simulink model "LQRAirrefuelingYingHu_full2Model"  (R2013a)
settings: Solver=ode45  StartTime=0.0  StopTime=100  RelTol=1e-3
values from neighbouring files (symbols this model uses):
  A_full = [A_full(1:7,1:7),zeros(7,1),A_full(1:7,8:11) ... (first row only)    [LQR_Calc2_F16YingHu_lonAndLa.m]
  B_full = [zeros(1,4);B(1:6,1:4);zeros(1,4);B(7:10,1:4)]    [LQR_Calc2_F16YingHu_lonAndLa.m]
  C_xd_h_yd = [C_xd_h,zeros(2,5) ... (first row only)    [LQR_Calc2_F16YingHu_lonAndLa.m]
  Ki = [Ki_lon,zeros(2,1) ... (first row only)    [LQR_Calc2_F16YingHu_lonAndLa.m]
  Kp = [Kp_lon,zeros(2,5) ... (first row only)    [LQR_Calc2_F16YingHu_lonAndLa.m]
undefined symbols (not defined in the file or in its folder): W_full
libraries: simulink x3
settings Model: Creator=Dai  LastModifiedBy=Dai

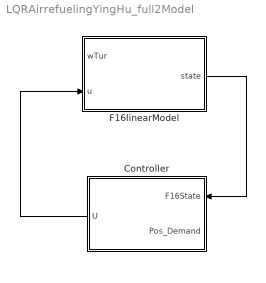
== system LQRAirrefuelingYingHu_full2Model ==
  Controller : Subsystem
  F16linearModel : Subsystem
  wires:
  F16linearModel/1(state) -> Controller/1(F16State)
  Controller/1(U) -> F16linearModel/2(u)

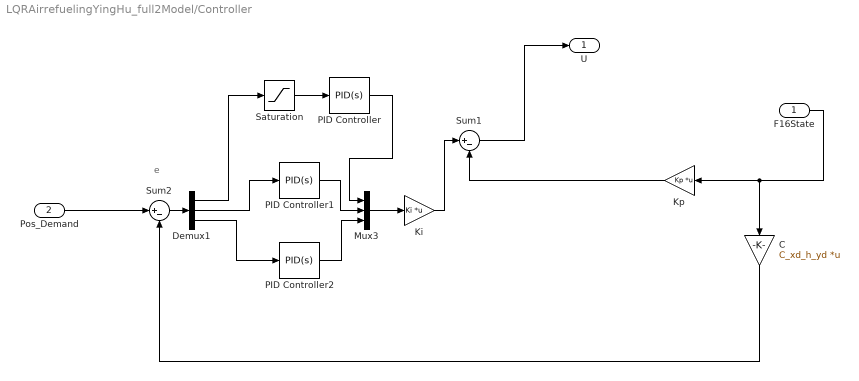
== system LQRAirrefuelingYingHu_full2Model/Controller ==
  note: e
  F16State : Inport
  Pos_Demand : Inport  Port=2
  C : Gain  Gain=C_xd_h_yd  Multiplication=Matrix(K*u) (u vector)
  Demux1 : Demux  Outputs=3
  Ki : Gain  Gain=Ki  Multiplication=Matrix(K*u) (u vector)
  Kp : Gain  Gain=Kp  Multiplication=Matrix(K*u) (u vector)
  Mux3 : Mux  Inputs=3
  PID Controller : simulink/Continuous/PID Controller  Controller=PID  TimeDomain=Continuous-time  SampleTime=1  IntegratorMethod=Forward Euler  FilterMethod=Forward Euler  Form=Parallel  P=0  I=1.2  D=0  N=100  InitialConditionSource=internal  InitialConditionForIntegrator=0  InitialConditionForFilter=0  ExternalReset=none  LimitOutput=off  UpperSaturationLimit=inf  LowerSaturationLimit=-inf  LinearizeAsGain=on  AntiWindupMode=none  Kb=1  TrackingMode=off  Kt=1  PParamMin=[]  PParamMax=[]  IParamMin=[]  IParamMax=[]  DParamMin=[]  DParamMax=[]  NParamMin=[]  NParamMax=[]  KbParamMin=[]  KbParamMax=[]  KtParamMin=[]  KtParamMax=[]  POutMin=[]  POutMax=[]  IOutMin=[]  IOutMax=[]  DOutMin=[]  DOutMax=[]  NOutMin=[]  NOutMax=[]  KbOutMin=[]  KbOutMax=[]  KtOutMin=[]  KtOutMax=[]  IntegratorOutMin=[]  IntegratorOutMax=[]  FilterOutMin=[]  FilterOutMax=[]  SumOutMin=[]  SumOutMax=[]  SumI1OutMin=[]  SumI1OutMax=[]  SumI2OutMin=[]  SumI2OutMax=[]  SumI3OutMin=[]  SumI3OutMax=[]  SumDOutMin=[]  SumDOutMax=[]  SaturationOutMin=[]  SaturationOutMax=[]  IntegratorContinuousStateAttributes=''  IntegratorStateMustResolveToSignalObject=off  IntegratorRTWStateStorageClass=Auto  FilterContinuousStateAttributes=''  FilterStateMustResolveToSignalObject=off  FilterRTWStateStorageClass=Auto
  PID Controller1 : simulink/Continuous/PID Controller  Controller=PID  TimeDomain=Continuous-time  SampleTime=1  IntegratorMethod=Forward Euler  FilterMethod=Forward Euler  Form=Parallel  P=0  I=1.5  D=0  N=100  InitialConditionSource=internal  InitialConditionForIntegrator=0  InitialConditionForFilter=0  ExternalReset=none  LimitOutput=off  UpperSaturationLimit=inf  LowerSaturationLimit=-inf  LinearizeAsGain=on  AntiWindupMode=none  Kb=1  TrackingMode=off  Kt=1  PParamMin=[]  PParamMax=[]  IParamMin=[]  IParamMax=[]  DParamMin=[]  DParamMax=[]  NParamMin=[]  NParamMax=[]  KbParamMin=[]  KbParamMax=[]  KtParamMin=[]  KtParamMax=[]  POutMin=[]  POutMax=[]  IOutMin=[]  IOutMax=[]  DOutMin=[]  DOutMax=[]  NOutMin=[]  NOutMax=[]  KbOutMin=[]  KbOutMax=[]  KtOutMin=[]  KtOutMax=[]  IntegratorOutMin=[]  IntegratorOutMax=[]  FilterOutMin=[]  FilterOutMax=[]  SumOutMin=[]  SumOutMax=[]  SumI1OutMin=[]  SumI1OutMax=[]  SumI2OutMin=[]  SumI2OutMax=[]  SumI3OutMin=[]  SumI3OutMax=[]  SumDOutMin=[]  SumDOutMax=[]  SaturationOutMin=[]  SaturationOutMax=[]  IntegratorContinuousStateAttributes=''  IntegratorStateMustResolveToSignalObject=off  IntegratorRTWStateStorageClass=Auto  FilterContinuousStateAttributes=''  FilterStateMustResolveToSignalObject=off  FilterRTWStateStorageClass=Auto
  PID Controller2 : simulink/Continuous/PID Controller  Controller=PID  TimeDomain=Continuous-time  SampleTime=1  IntegratorMethod=Forward Euler  FilterMethod=Forward Euler  Form=Parallel  P=0  I=1  D=0  N=100  InitialConditionSource=internal  InitialConditionForIntegrator=0  InitialConditionForFilter=0  ExternalReset=none  LimitOutput=off  UpperSaturationLimit=inf  LowerSaturationLimit=-inf  LinearizeAsGain=on  AntiWindupMode=none  Kb=1  TrackingMode=off  Kt=1  PParamMin=[]  PParamMax=[]  IParamMin=[]  IParamMax=[]  DParamMin=[]  DParamMax=[]  NParamMin=[]  NParamMax=[]  KbParamMin=[]  KbParamMax=[]  KtParamMin=[]  KtParamMax=[]  POutMin=[]  POutMax=[]  IOutMin=[]  IOutMax=[]  DOutMin=[]  DOutMax=[]  NOutMin=[]  NOutMax=[]  KbOutMin=[]  KbOutMax=[]  KtOutMin=[]  KtOutMax=[]  IntegratorOutMin=[]  IntegratorOutMax=[]  FilterOutMin=[]  FilterOutMax=[]  SumOutMin=[]  SumOutMax=[]  SumI1OutMin=[]  SumI1OutMax=[]  SumI2OutMin=[]  SumI2OutMax=[]  SumI3OutMin=[]  SumI3OutMax=[]  SumDOutMin=[]  SumDOutMax=[]  SaturationOutMin=[]  SaturationOutMax=[]  IntegratorContinuousStateAttributes=''  IntegratorStateMustResolveToSignalObject=off  IntegratorRTWStateStorageClass=Auto  FilterContinuousStateAttributes=''  FilterStateMustResolveToSignalObject=off  FilterRTWStateStorageClass=Auto
  Saturation : Saturate
  Sum1 : Sum  Inputs=|+-
  Sum2 : Sum  Inputs=|+-
  U : Outport
  wires:
  Sum2/1 -> Demux1/1
  Kp/1 -> Sum1/2
  Ki/1 -> Sum1/1
  C/1 -> Sum2/2
  Pos_Demand/1 -> Sum2/1
  Mux3/1 -> Ki/1
  Sum1/1 -> U/1
  Demux1/1 -> Saturation/1
  Demux1/2 -> PID Controller1/1
  F16State/1 -> Kp/1, C/1
  PID Controller1/1 -> Mux3/2
  Saturation/1 -> PID Controller/1
  PID Controller/1 -> Mux3/1
  Demux1/3 -> PID Controller2/1
  PID Controller2/1 -> Mux3/3

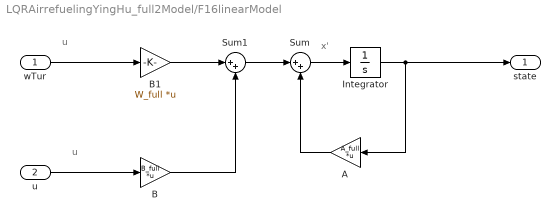
== system LQRAirrefuelingYingHu_full2Model/F16linearModel ==
  note: x'
  note: u
  note: u
  wTur : Inport
  u : Inport  Port=2
  A : Gain  Gain=A_full  Multiplication=Matrix(K*u) (u vector)
  B : Gain  Gain=B_full  Multiplication=Matrix(K*u) (u vector)
  B1 : Gain  Gain=W_full  Multiplication=Matrix(K*u) (u vector)
  Integrator : Integrator
  Sum : Sum  Inputs=|++
  Sum1 : Sum  Inputs=|++
  state : Outport
  wires:
  u/1 -> B/1
  Sum/1 -> Integrator/1
  Integrator/1 -> state/1, A/1
  wTur/1 -> B1/1
  A/1 -> Sum/2
  B/1 -> Sum1/2
  Sum1/1 -> Sum/1
  B1/1 -> Sum1/1
